simulink model "BBBL_Test2"  (R2017a)
settings: Solver=FixedStepDiscrete  StartTime=0.0  StopTime=60.0  RelTol=1e-3  EnableMultiTasking=on
libraries: simulink x3
settings Model: ExtModeTrigDuration=2  Creator=gcampa  LastModifiedBy=Parker
settings SolverCC: PositivePriorityOrder=on
settings DataIOCC: SaveFormat=Array  SignalLogging=off  DSMLogging=off
settings OptimizationCC: MaxStackSize=64
settings DebuggingCC: SolverPrmCheckMsg=warning  ParameterTunabilityLossMsg=error  AllowSymbolicDim=off  SFUnexpectedBacktrackingDiag=warning  SFNoUnconditionalDefaultTransitionDiag=warning  SFExecutionAtInitializationDiag=none
settings HardwareCC: ProdBitPerPointer=32  ProdBitPerSizeT=32  ProdBitPerPtrDiffT=32  ProdLargestAtomicInteger=Long  ProdLargestAtomicFloat=Double  ProdWordSize=32  ProdHWDeviceType=ARM Compatible->ARM Cortex
settings ModelReferenceCC: PropagateSignalLabelsOutOfModel=off
settings SFSimCC: MATLABDynamicMemAlloc=off
settings RTWCC: SystemTargetFile=ert.tlc  HardwareBoard=Raspberry Pi  TLCOptions="-aInlineSetEventsForThisBaseRateFcn=TLC_FALSE -aSuppressMultiTaskScheduler=TLC_FALSE  -aRateBasedStepFcn=0"  TemplateMakefile=ert_default_tmf  Description=Embedded Coder  Toolchain=GNU GCC Raspberry Pi  BuildConfiguration=Faster Runs
settings CodeAppCC: ForceParamTrailComments=on  IgnoreCustomStorageClasses=off  OperatorAnnotations=on  SimulinkDataObjDesc=on  SFDataObjDesc=on  MATLABFcnDesc=on  InsertBlockDesc=on  MATLABSourceComments=on
settings ERTTargetCC: MultiwordLength=2048  SupportVariableSizeSignals=on
settings ConfigComp: CovMetricSettings=dw  CovHtmlReporting=on  CovSaveCumulativeToWorkspaceVar=on  CovSaveSingleToWorkspaceVar=on  CovExternalEMLEnable=off  CovSFcnEnable=off

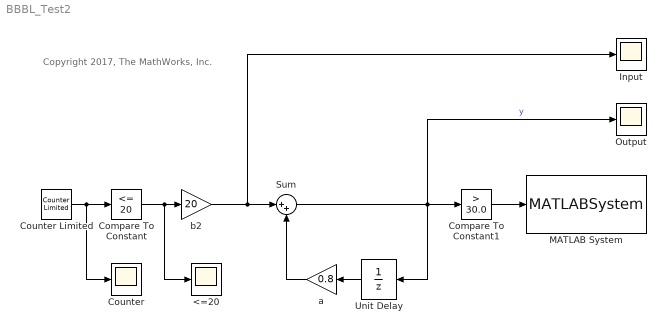
== system BBBL_Test2 ==
  note: Copyright 2017, The MathWorks, Inc.
  <=20 : Scope
  Compare To Constant : simulink/Logic and Bit Operations/Compare To Constant  relop=<=  const=20  OutDataTypeStr=uint8
  Compare To Constant1 : simulink/Logic and Bit Operations/Compare To Constant  relop=>  const=30.0  OutDataTypeStr=uint8
  Counter : Scope
  Counter Limited : simulink/Sources/Counter Limited  uplimit=40  tsamp=0.1
  Input : Scope
  MATLAB System : MATLABSystem  System=rc_blink_sys  rc_led_t=1
      mask Type: rc_blink_sys
      mask Display:
      | disp('rc_blink_sys');
      | port_label('input',1,'u');
  Output : Scope
  Sum : Sum  Inputs=|++
  Unit Delay : UnitDelay  SampleTime=-1
  a : Gain  Gain=0.8  SaturateOnIntegerOverflow=on  OutDataTypeStr=Inherit: Same as input  ParamDataTypeStr=Inherit: Same as input
  b2 : Gain  Gain=20  ParamDataTypeStr=double  OutDataTypeStr=double  SaturateOnIntegerOverflow=on
  wires:
  a/1 -> Sum/2
  Unit Delay/1 -> a/1
  Sum/1 -> Unit Delay/1, Output/1, Compare To Constant1/1  "y"
  Counter Limited/1 -> Counter/1, Compare To Constant/1
  Compare To Constant/1 -> <=20/1, b2/1
  b2/1 -> Input/1, Sum/1
  Compare To Constant1/1 -> MATLAB System/1
